simulink model "t6_3_Vectorizacion"  (R2024a)
settings: Solver=FixedStepAuto  StartTime=0.0  StopTime=20  FixedStep=.01  RelTol=1e-3
InitFcn:
  | rho=0.074;
  | Cd=0.67;
  | A=0.2;
  | v0=30;
  | theta0=pi/6;
StopFcn:
  | %data = [out.tout,out.x,out.y];
  | %save('EmpriricalData.mat','data')
settings Model: Creator=scpmoxxa  LastModifiedBy=scpmoxxa
settings OptimizationCC: ReuseModelBlockBuffer=off
settings DebuggingCC: UnconnectedInputMsg=warning  UnconnectedOutputMsg=warning  UnconnectedLineMsg=warning
settings ModelReferenceCC: EnableRefExpFcnMdlSchedulingChecks=on
settings RTWCC: GPUComputeCapability=3.5  DLArmComputeVersion=19.05

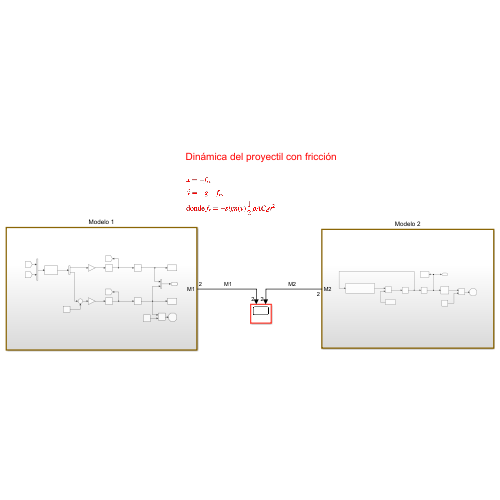
[thumbnail: Simulink's stored preview of the top-level diagram]
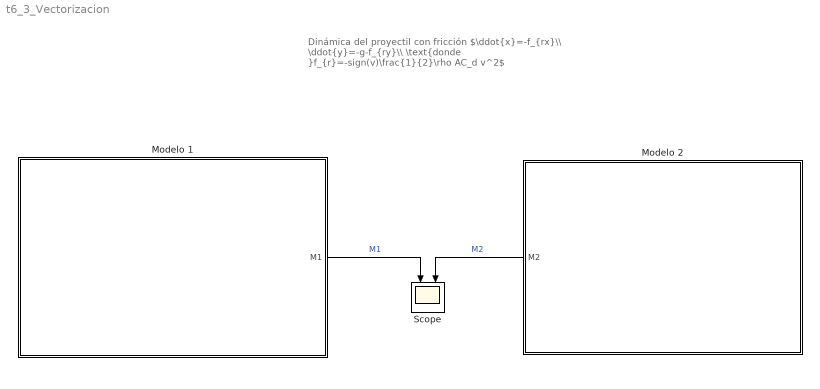
== system t6_3_Vectorizacion ==
  note: Dinámica del proyectil con fricción
      |
      | $\ddot{x}=-f_{rx}\\ \ddot{y}=-g-f_{ry}\\ \text{donde }f_{r}=-sign(v)\frac{1}{2}\rho AC_d v^2$
  Modelo 1 : Subsystem
  Modelo 2 : Subsystem
  Scope : Scope  NumInputPorts=2
  wires:
  Modelo 1/1(M1) -> Scope/1  "M1"
  Modelo 2/1(M2) -> Scope/2  "M2"

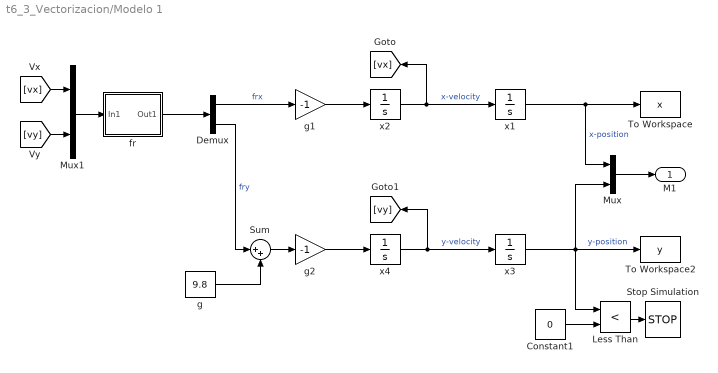
== system t6_3_Vectorizacion/Modelo 1 ==
  Constant1 : Constant  Value=0
  Demux : Demux  Outputs=2
  Less Than : RelationalOperator  Operator=<  OutDataTypeStr=boolean  RndMeth=Simplest  InputSameDT=off
  Mux : Mux  Inputs=2
  Mux1 : Mux  Inputs=2
  Stop Simulation : Stop
  Sum : Sum  Inputs=|++
  To Workspace : ToWorkspace  VariableName=x  SampleTime=-1
  To Workspace2 : ToWorkspace  VariableName=y  SampleTime=-1
  fr : Subsystem  TreatAsAtomicUnit=on
  g : Constant  Value=9.8
  g1 : Gain  Gain=-1
  g2 : Gain  Gain=-1
  x1 : Integrator
      settings: AttributesFormatString=x10= %<InitialCondition>
  x2 : Integrator  InitialCondition=v0*cos(theta0)
      settings: AttributesFormatString=x20= %<InitialCondition>
  x3 : Integrator  InitialCondition=20
      settings: AttributesFormatString=x30= %<InitialCondition>
  x4 : Integrator  InitialCondition=v0*sin(theta0)
      settings: AttributesFormatString=x40= %<InitialCondition>
  M1 : Outport
  wires:
  g/1 -> Sum/2
  x4/1 -> [vy], x3/1  "y-velocity"
  Less Than/1 -> Stop Simulation/1
  fr/1(Out1) -> Demux/1
  g1/1 -> x2/1
  x2/1 -> [vx], x1/1  "x-velocity"
  x3/1 -> Mux/2, Less Than/1, To Workspace2/1  "y-position"
  x1/1 -> Mux/1, To Workspace/1  "x-position"
  Demux/2 -> Sum/1  "fry"
  Demux/1 -> g1/1  "frx"
  Constant1/1 -> Less Than/2
  [vx] -> Mux1/1
  g2/1 -> x4/1
  Sum/1 -> g2/1
  Mux1/1 -> fr/1(In1)
  [vy] -> Mux1/2
  Mux/1 -> M1/1

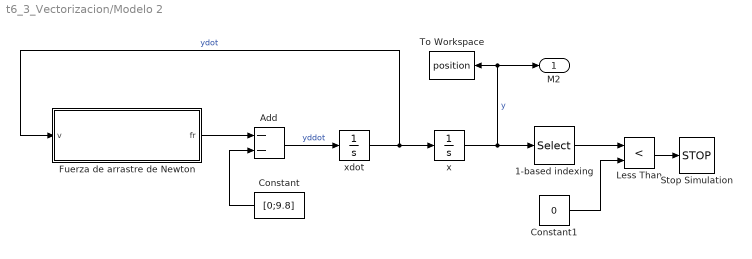
== system t6_3_Vectorizacion/Modelo 2 ==
  1-based indexing : Selector  InputPortWidth=2  IndexOptions=Index vector (dialog)  Indices=2  OutputSizes=1
  Add : Sum  Inputs=--
  Constant : Constant  Value=[0;9.8]
  Constant1 : Constant  Value=0
  Fuerza de arrastre de Newton : Subsystem
  Less Than : RelationalOperator  Operator=<  OutDataTypeStr=boolean  RndMeth=Simplest  InputSameDT=off
  Stop Simulation : Stop
  To Workspace : ToWorkspace  VariableName=position  SampleTime=-1
  x : Integrator  InitialCondition=[0;20]
  xdot : Integrator  InitialCondition=[v0*cos(theta0);v0*sin(theta0)]
  M2 : Outport
  wires:
  xdot/1 -> x/1, Fuerza de arrastre de Newton/1(v)  "ydot"
  Fuerza de arrastre de Newton/1(fr) -> Add/1
  1-based indexing/1 -> Less Than/1
  x/1 -> M2/1, To Workspace/1, 1-based indexing/1  "y"
  Constant/1 -> Add/2
  Add/1 -> xdot/1  "yddot"
  Constant1/1 -> Less Than/2
  Less Than/1 -> Stop Simulation/1

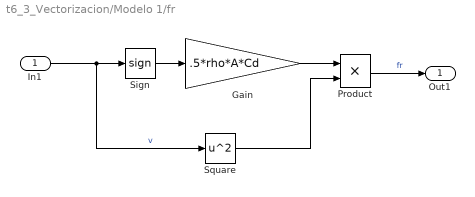
== system t6_3_Vectorizacion/Modelo 1/fr ==
  In1 : Inport
  Gain : Gain  Gain=.5*rho*A*Cd
  Product : Product
  Sign : Signum
  Square : Math  Operator=square
  Out1 : Outport
  wires:
  Square/1 -> Product/2
  In1/1 -> Square/1, Sign/1  "v"
  Gain/1 -> Product/1
  Product/1 -> Out1/1  "fr"
  Sign/1 -> Gain/1

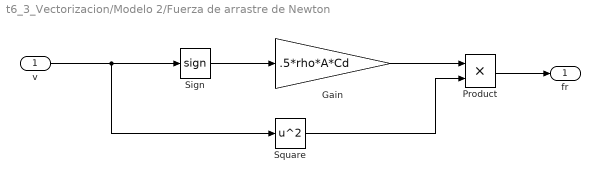
== system t6_3_Vectorizacion/Modelo 2/Fuerza de arrastre de Newton ==
  v : Inport
  Gain : Gain  Gain=.5*rho*A*Cd
  Product : Product
  Sign : Signum
  Square : Math  Operator=square
  fr : Outport
  wires:
  Square/1 -> Product/2
  v/1 -> Square/1, Sign/1
  Gain/1 -> Product/1
  Product/1 -> fr/1
  Sign/1 -> Gain/1
